simulink model "chap14_3sim"  (Simulink 7.7)
settings: Solver=ode45  StartTime=0.0  StopTime=10.0  FixedStep=0.002  RelTol=1e-3
settings Model: Creator=liujk  LastModifiedBy=ljk
settings DataIOCC: SignalLoggingName=sigsOut
settings OptimizationCC: ExpressionDepthLimit=128
settings DebuggingCC: SaveWithParameterizedLinksMsg=none  SignalResolutionControl=TryResolveAllWithWarning  SolverPrmCheckMsg=none  MultiTaskDSMMsg=warning  MultiTaskCondExecSysMsg=none  StrictBusMsg=None
settings HardwareCC: TargetUnknown=on
settings RTWCC: IncludeERTFirstTime=on
settings CodeAppCC: CustomSymbolStrType=$N$R$M_T

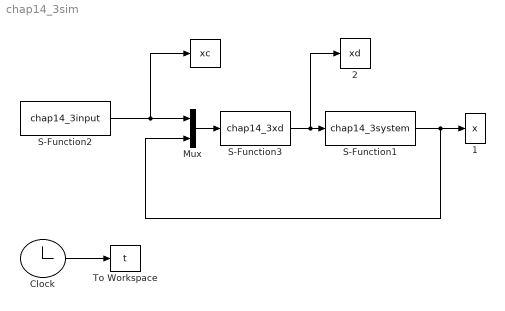
== system chap14_3sim ==
  "  " : ToWorkspace  VariableName=xc  SampleTime=-1  SaveFormat=Array
  "  1" : ToWorkspace  VariableName=x  SampleTime=-1  SaveFormat=Array
  "  2" : ToWorkspace  VariableName=xd  SampleTime=-1  SaveFormat=Array
  Clock : Clock
      settings: Decimation=10
  Mux : Mux  Inputs=2
  S-Function1 : S-Function  FunctionName=chap14_3system  EnableBusSupport=off
  S-Function2 : S-Function  FunctionName=chap14_3input  EnableBusSupport=off
  S-Function3 : S-Function  FunctionName=chap14_3xd  EnableBusSupport=off
  To Workspace : ToWorkspace  VariableName=t  SampleTime=-1  SaveFormat=Array
  wires:
  S-Function1/1 -> "  1"/1, Mux/2
  Clock/1 -> To Workspace/1
  S-Function3/1 -> S-Function1/1, "  2"/1
  S-Function2/1 -> Mux/1, "  "/1
  Mux/1 -> S-Function3/1
